simulink model "expt_5_a"  (R2018b)
settings: Solver=VariableStepAuto  StartTime=0.0  StopTime=0.5  MaxStep=1e-4  RelTol=1e-4
settings Model: Creator=sangh  LastModifiedBy=sangh

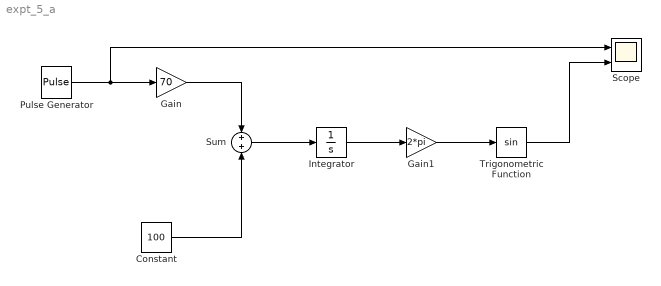
== system expt_5_a ==
  Constant : Constant  Value=100
  Gain : Gain  Gain=70
  Gain1 : Gain  Gain=2*pi
  Integrator : Integrator
  Pulse Generator : DiscretePulseGenerator  PulseType=Time based  Period=0.1  PulseWidth=50
  Scope : Scope  NumInputPorts=2
  Sum : Sum
  Trigonometric Function : Trigonometry
  wires:
  Pulse Generator/1 -> Scope/1, Gain/1
  Gain/1 -> Sum/1
  Constant/1 -> Sum/2
  Sum/1 -> Integrator/1
  Integrator/1 -> Gain1/1
  Gain1/1 -> Trigonometric Function/1
  Trigonometric Function/1 -> Scope/2
